simulink model "perturbacao"  (R2022b)
settings: Solver=VariableStepAuto  StartTime=0.0  StopTime=10.0  RelTol=1e-3
settings Model: Creator=vfton  LastModifiedBy=matak
settings ModelReferenceCC: EnableRefExpFcnMdlSchedulingChecks=on

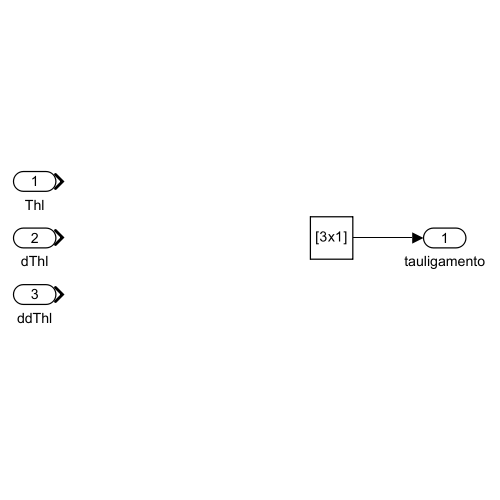
[thumbnail: Simulink's stored preview of the top-level diagram]
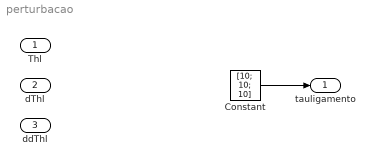
== system perturbacao ==
  Thl : Inport  PortDimensions=3
  dThl : Inport  Port=2  PortDimensions=3
  ddThl : Inport  Port=3  PortDimensions=3
  Constant : Constant  Value=[10; 10; 10]  VectorParams1D=off
  tauligamento : Outport
  wires:
  Constant/1 -> tauligamento/1
